simulink model "RCV_Tune"  (R2020b)
settings: Solver=VariableStepAuto  StartTime=0.0  StopTime=10  MaxStep=0.001  RelTol=1e-3  AbsTol=1e-3
model workspace (MAT data in the model file):
  O2 = 0.543892545144
  O2_conc = 0.301567785759
  v_area = 1
libraries: fl_lib x5, nesl_utility x4, pid_lib x1
(part 2 of 2)

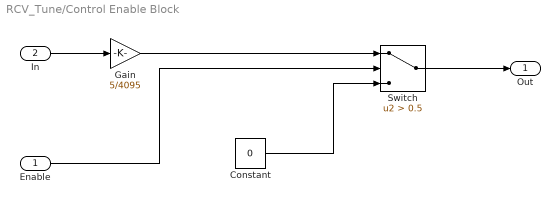
== system RCV_Tune/Control Enable Block ==
  Enable : Inport
  In : Inport  Port=2
  Constant : Constant  Value=0
  Gain : Gain  Gain=5/4095
  Switch : Switch  Criteria=u2 > Threshold  Threshold=0.5
  Out : Outport
  wires:
  Enable/1 -> Switch/2
  In/1 -> Gain/1
  Switch/1 -> Out/1
  Constant/1 -> Switch/3
  Gain/1 -> Switch/1

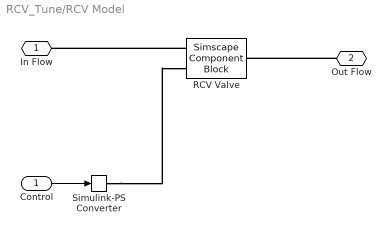
== system RCV_Tune/RCV Model ==
  Control : Inport
  RCV Valve : SimscapeComponentBlock  SourceFile=rcv_exhale_volt_pr_flow_lookup  ComponentPath=rcv_exhale_volt_pr_flow_lookup  ComponentVariants="[\"rcv_exhale_volt_pr_flow_lookup\"]"  ComponentVariantNames="[\"rcv_exhale_volt_pr_flow_lookup\"]"  ClassName=rcv_exhale_volt_pr_flow_lookup  SchemaVersion=1  rho_nominal=0 kg/m^3  area=0.01 m^2  laminar_fraction=1e-3
      settings: CopyFcn=simscape.engine.sli.internal.componentblockcallback(gcbh,'COPY')  PreCopyFcn=simscape.engine.sli.internal.componentblockcallback(gcbh,'PRECOPY')  PreDeleteFcn=simscape.engine.sli.internal.componentblockcallback(gcbh,'PREDELETE')  InternalSimscapePortConfiguration="{\"Bottom\":[],\"Left\":[{\"id\":\"A\",\"label\":\"A\",\"type\":\"foundation.gas.gas\"},{\"id\":\"v_posin\",\"label\":\"v_posin\",\"type\":\"input\"}],\"Right\":[{\"id\":\"B\",\"label\":\"B\",\"type\":\"foundation.gas.gas\"}],\"Top\":[]}"
      mask Type: RCV_Exhale Valve for Ventilator (G)
  Simulink-PS Converter : nesl_utility/Simulink-PS Converter  PhysicalDomain=network_engine_domain  SubClassName=ps_input  LeftPortType=input  RightPortType=output  PseudoPeriodic=off  Frequencies=[]  NoiseDistribution=none  NoiseParameters=[]  Unit=1  AffineConversion=off  FilteringAndDerivatives=provide  SimscapeFilterOrder=1  InputFilterTimeConstant=0.001  UdotUserProvided=0
  In Flow : PMIOPort  Side=Left
  Out Flow : PMIOPort  Port=2  Side=Right
  wires:
  Control/1 -> Simulink-PS Converter/1
  connections:
  Simulink-PS Converter/RConn1 -- RCV Valve/LConn2
  RCV Valve/LConn1 -- In Flow/RConn1
  Out Flow/RConn1 -- RCV Valve/RConn1
